simulink model "gm_zynqRadioHWSWAXI4StreamAD9361AD9364SL"  (R2024b)
settings: Solver=FixedStepDiscrete  StartTime=0.0  StopTime=18000/Fs  RelTol=1e-3
PreLoadFcn:
  | Fs = 3840000;
  | nsamp = 4096;
  | t = (0:nsamp)/Fs;
  | y = chirp(t(1:2048),0,t(2048),Fs/20,[],90);
  | ly = length(y);
InitFcn:
  | Fs = 3840000;
  | nsamp = 4096;
  | t = (0:nsamp)/Fs;
  | y = chirp(t(1:2048),0,t(2048),Fs/20,[],90);
  | ly = length(y);
libraries: hdlsllib x11, simulink x4, dspsrcs4 x2, sdrzblksprivate x1
settings Model: Creator=The MathWorks, Inc.  LastModifiedBy=daniel
settings SolverCC: AlgebraicLoopSolver=TrustRegion
settings OptimizationCC: BlockReduction=off  ConditionallyExecuteInputs=off  DefaultParameterBehavior=Inlined
settings DebuggingCC: AlgebraicLoopMsg=error  InheritedTsInSrcMsg=none  UnconnectedInputMsg=warning  UnconnectedOutputMsg=warning  UnconnectedLineMsg=warning
settings HardwareCC: ProdBitPerPointer=32  ProdBitPerSizeT=32  ProdBitPerPtrDiffT=32  ProdLargestAtomicFloat=None  ProdIntDivRoundTo=Undefined  ProdEndianess=Unspecified  ProdWordSize=32  ProdHWDeviceType=ASIC/FPGA->ASIC/FPGA  TargetBitPerLong=64  TargetBitPerPointer=64  TargetBitPerSizeT=64  TargetBitPerPtrDiffT=64  TargetLongLongMode=on  TargetIntDivRoundTo=Zero  TargetEndianess=LittleEndian  TargetWordSize=64  TargetHWDeviceType=Custom Processor->MATLAB Host Computer  ProdEqTarget=off
settings ModelReferenceCC: EnableRefExpFcnMdlSchedulingChecks=on
settings RTWCC: GPUComputeCapability=3.5

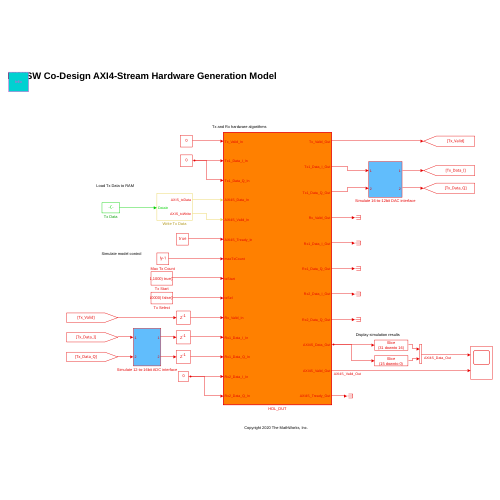
[thumbnail: Simulink's stored preview of the top-level diagram]
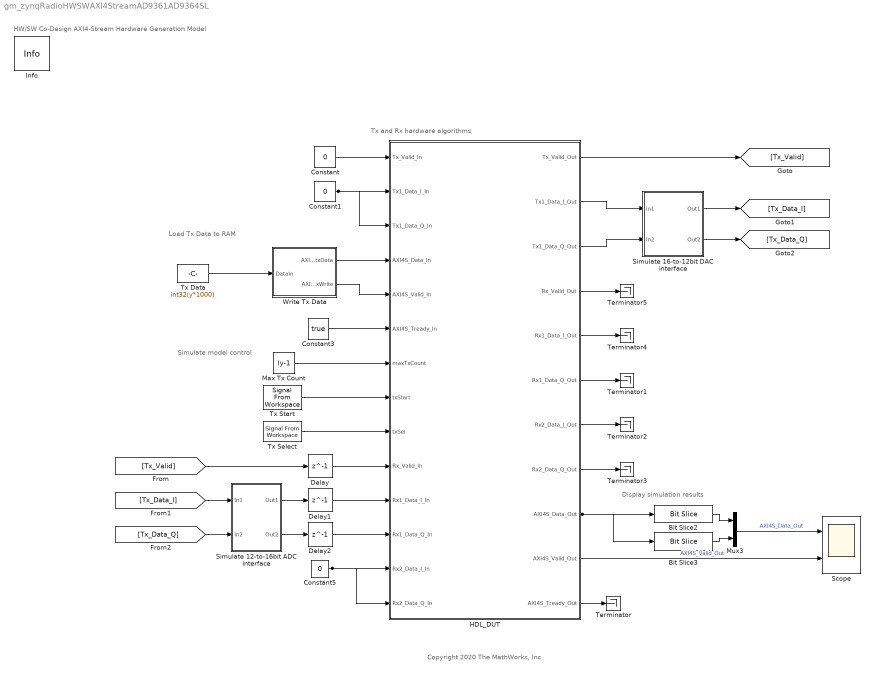
== system gm_zynqRadioHWSWAXI4StreamAD9361AD9364SL ==
  note: Copyright 2020 The MathWorks, Inc.
  note: HW/SW Co-Design AXI4-Stream Hardware Generation Model
  note: Load Tx Data to RAM
  note: Display simulation results
  note: Simulate model control
  note: Tx and Rx hardware algorithms
  Bit Slice2 : hdlsllib/Logic and Bit Operations/Bit Slice  lidx=31  ridx=16
  Bit Slice3 : hdlsllib/Logic and Bit Operations/Bit Slice  lidx=15  ridx=0
  Constant : Constant  Value=0  OutDataTypeStr=boolean  SampleTime=-1
  Constant1 : Constant  Value=0  OutDataTypeStr=int16  SampleTime=-1
  Constant3 : Constant  Value=true  SampleTime=-1
  Constant5 : Constant  Value=0  OutDataTypeStr=int16  SampleTime=-1
  Delay : Delay  DelayLength=1
  Delay1 : Delay  DelayLength=1
  Delay2 : Delay  DelayLength=1
  HDL_DUT : Subsystem  TreatAsAtomicUnit=on
  Info : sdrzblksprivate/Info  SystemSampleTime=-1  VariantActivationTime=update diagram  AllowFlexibleInterface=on  Latency=0  AutoFrameSizeCalculation=off
  Max Tx Count : Constant  Value=ly-1  OutDataTypeStr=int16  SampleTime=-1
  Mux3 : Mux  Inputs=2
  Scope : Scope  NumInputPorts=2
  Simulate 12-to-16bit ADC interface : Subsystem
  Simulate 16-to-12bit DAC interface : Subsystem
  Terminator{,1..5} (6 alike) : Terminator
  Tx Data : Constant  Value=int32(y*1000)  OutDataTypeStr=int32  SampleTime=-1
  Tx Select : dspsrcs4/Signal From Workspace  X=[true(1,10000) false(1,1000)]  Ts=1/Fs  nsamps=1  OutputAfterFinalValue=Holding final value  ignoreOrWarnInputAndFrameLengths=off  OutputFrames=off
  Tx Start : dspsrcs4/Signal From Workspace  X=[false(1,7000) true(1,100) false(1,1000) true(1,100) false(1,2000) true(1,100)]  Ts=1/Fs  nsamps=1  OutputAfterFinalValue=Setting to zero  ignoreOrWarnInputAndFrameLengths=off  OutputFrames=off
  Write Tx Data : Subsystem
  wires:
  HDL_DUT/4(Rx_Valid_Out) -> Terminator5/1
  HDL_DUT/5(Rx1_Data_I_Out) -> Terminator4/1
  HDL_DUT/8(Rx2_Data_Q_Out) -> Terminator3/1
  HDL_DUT/7(Rx2_Data_I_Out) -> Terminator2/1
  HDL_DUT/6(Rx1_Data_Q_Out) -> Terminator1/1
  Mux3/1 -> Scope/1  "AXI4S_Data_Out"
  Bit Slice3/1 -> Mux3/2
  Tx Data/1 -> Write Tx Data/1(DataIn)
  HDL_DUT/11(AXI4S_Tready_Out) -> Terminator/1
  Constant3/1 -> HDL_DUT/6(AXI4S_Tready_In)
  Simulate 12-to-16bit ADC interface/2(Out2) -> Delay2/1
  Simulate 12-to-16bit ADC interface/1(Out1) -> Delay1/1
  [Tx_Data_Q] -> Simulate 12-to-16bit ADC interface/2(In2)
  [Tx_Data_I] -> Simulate 12-to-16bit ADC interface/1(In1)
  Simulate 16-to-12bit DAC interface/2(Out2) -> [Tx_Data_Q]
  Simulate 16-to-12bit DAC interface/1(Out1) -> [Tx_Data_I]
  HDL_DUT/3(Tx1_Data_Q_Out) -> Simulate 16-to-12bit DAC interface/2(In2)
  HDL_DUT/2(Tx1_Data_I_Out) -> Simulate 16-to-12bit DAC interface/1(In1)
  HDL_DUT/9(AXI4S_Data_Out) -> Bit Slice2/1, Bit Slice3/1
  Delay/1 -> HDL_DUT/10(Rx_Valid_In)
  HDL_DUT/10(AXI4S_Valid_Out) -> Scope/2  "AXI4S_Valid_Out"
  Max Tx Count/1 -> HDL_DUT/7(maxTxCount)
  Tx Select/1 -> HDL_DUT/9(txSel)
  Tx Start/1 -> HDL_DUT/8(txStart)
  Write Tx Data/2(AXIS_txWrite) -> HDL_DUT/5(AXI4S_Valid_In)
  Constant5/1 -> HDL_DUT/14(Rx2_Data_Q_In), HDL_DUT/13(Rx2_Data_I_In)
  Constant1/1 -> HDL_DUT/3(Tx1_Data_Q_In), HDL_DUT/2(Tx1_Data_I_In)
  Write Tx Data/1(AXIS_txData) -> HDL_DUT/4(AXI4S_Data_In)
  Delay2/1 -> HDL_DUT/12(Rx1_Data_Q_In)
  Constant/1 -> HDL_DUT/1(Tx_Valid_In)
  HDL_DUT/1(Tx_Valid_Out) -> [Tx_Valid]
  Delay1/1 -> HDL_DUT/11(Rx1_Data_I_In)
  Bit Slice2/1 -> Mux3/1
  [Tx_Valid] -> Delay/1

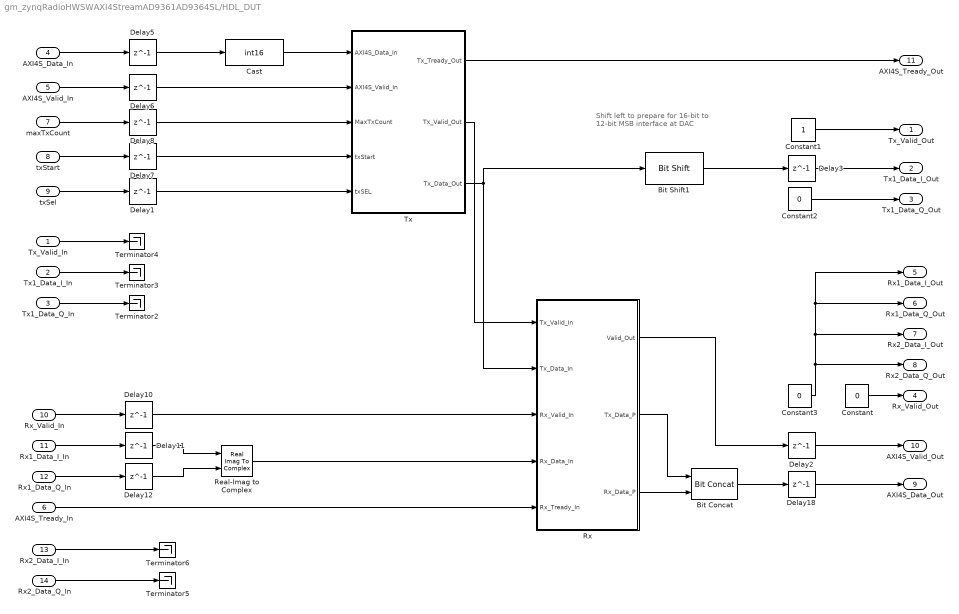
== system gm_zynqRadioHWSWAXI4StreamAD9361AD9364SL/HDL_DUT ==
  note: Shift left to prepare for 16-bit to 12-bit MSB interface at DAC
  Tx_Valid_In : Inport
  Tx1_Data_I_In : Inport  Port=2
  Tx1_Data_Q_In : Inport  Port=3
  AXI4S_Data_In : Inport  Port=4
  AXI4S_Valid_In : Inport  Port=5
  AXI4S_Tready_In : Inport  Port=6
  maxTxCount : Inport  Port=7
  txStart : Inport  Port=8
  txSel : Inport  Port=9
  Rx_Valid_In : Inport  Port=10
  Rx1_Data_I_In : Inport  Port=11
  Rx1_Data_Q_In : Inport  Port=12
  Rx2_Data_I_In : Inport  Port=13
  Rx2_Data_Q_In : Inport  Port=14
  Bit Concat : hdlsllib/Logic and Bit Operations/Bit Concat  numInputs=2
  Bit Shift1 : hdlsllib/Logic and Bit Operations/Bit Shift  mode=Shift Left Logical  N=4
  Cast : DataTypeConversion  OutDataTypeStr=int16  ConvertRealWorld=Stored Integer (SI)  SaturateOnIntegerOverflow=off  RndMeth=Floor
  Constant : Constant  Value=0  OutDataTypeStr=boolean  SampleTime=-1
  Constant1 : Constant  OutDataTypeStr=boolean  SampleTime=-1
  Constant2 : Constant  Value=0  OutDataTypeStr=int16  SampleTime=-1
  Constant3 : Constant  Value=0  OutDataTypeStr=int16  SampleTime=-1
  Delay{1..3,5..8,10..12,18} (11 alike) : Delay  DelayLength=1
  Real-Imag to Complex : RealImagToComplex
  Rx : Subsystem
  Terminator{2..6} (5 alike) : Terminator
  Tx : Subsystem
  Tx_Valid_Out : Outport
  Tx1_Data_I_Out : Outport  Port=2
  Tx1_Data_Q_Out : Outport  Port=3
  Rx_Valid_Out : Outport  Port=4
  Rx1_Data_I_Out : Outport  Port=5
  Rx1_Data_Q_Out : Outport  Port=6
  Rx2_Data_I_Out : Outport  Port=7
  Rx2_Data_Q_Out : Outport  Port=8
  AXI4S_Data_Out : Outport  Port=9
  AXI4S_Valid_Out : Outport  Port=10
  AXI4S_Tready_Out : Outport  Port=11
  wires:
  Constant1/1 -> Tx_Valid_Out/1
  Constant/1 -> Rx_Valid_Out/1
  AXI4S_Tready_In/1 -> Rx/5(Rx_Tready_In)
  Tx/1(Tx_Tready_Out) -> AXI4S_Tready_Out/1
  Delay2/1 -> AXI4S_Valid_Out/1
  Rx/3(Rx_Data_P) -> Bit Concat/2
  Rx/2(Tx_Data_P) -> Bit Concat/1
  Bit Shift1/1 -> Delay3/1
  Delay18/1 -> AXI4S_Data_Out/1
  Bit Concat/1 -> Delay18/1
  Rx/1(Valid_Out) -> Delay2/1
  Real-Imag to Complex/1 -> Rx/4(Rx_Data_In)
  Delay10/1 -> Rx/3(Rx_Valid_In)
  Constant3/1 -> Rx2_Data_Q_Out/1, Rx2_Data_I_Out/1, Rx1_Data_I_Out/1, Rx1_Data_Q_Out/1
  Constant2/1 -> Tx1_Data_Q_Out/1
  Delay3/1 -> Tx1_Data_I_Out/1
  Tx/2(Tx_Valid_Out) -> Rx/1(Tx_Valid_In)
  Delay12/1 -> Real-Imag to Complex/2
  Delay11/1 -> Real-Imag to Complex/1
  Tx/3(Tx_Data_Out) -> Rx/2(Tx_Data_In), Bit Shift1/1
  Cast/1 -> Tx/1(AXI4S_Data_In)
  Delay5/1 -> Cast/1
  Rx1_Data_Q_In/1 -> Delay12/1
  Rx1_Data_I_In/1 -> Delay11/1
  Rx_Valid_In/1 -> Delay10/1
  Rx2_Data_I_In/1 -> Terminator6/1
  Rx2_Data_Q_In/1 -> Terminator5/1
  Delay1/1 -> Tx/5(txSEL)
  Delay8/1 -> Tx/3(MaxTxCount)
  Delay7/1 -> Tx/4(txStart)
  Delay6/1 -> Tx/2(AXI4S_Valid_In)
  txSel/1 -> Delay1/1
  maxTxCount/1 -> Delay8/1
  txStart/1 -> Delay7/1
  AXI4S_Valid_In/1 -> Delay6/1
  AXI4S_Data_In/1 -> Delay5/1
  Tx1_Data_Q_In/1 -> Terminator2/1
  Tx_Valid_In/1 -> Terminator4/1
  Tx1_Data_I_In/1 -> Terminator3/1

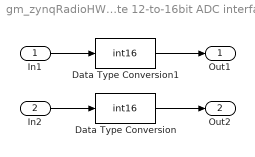
== system gm_zynqRadioHWSWAXI4StreamAD9361AD9364SL/Simulate 12-to-16bit ADC interface ==
  In1 : Inport
  In2 : Inport  Port=2
  Data Type Conversion : DataTypeConversion  OutDataTypeStr=int16  SaturateOnIntegerOverflow=off  RndMeth=Floor
  Data Type Conversion1 : DataTypeConversion  OutDataTypeStr=int16  SaturateOnIntegerOverflow=off  RndMeth=Floor
  Out1 : Outport
  Out2 : Outport  Port=2
  wires:
  Data Type Conversion/1 -> Out2/1
  In1/1 -> Data Type Conversion1/1
  Data Type Conversion1/1 -> Out1/1
  In2/1 -> Data Type Conversion/1

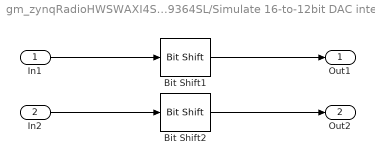
== system gm_zynqRadioHWSWAXI4StreamAD9361AD9364SL/Simulate 16-to-12bit DAC interface ==
  In1 : Inport
  In2 : Inport  Port=2
  Bit Shift1 : hdlsllib/Logic and Bit Operations/Bit Shift  mode=Shift Right Arithmetic  N=4
  Bit Shift2 : hdlsllib/Logic and Bit Operations/Bit Shift  mode=Shift Right Arithmetic  N=4
  Out1 : Outport
  Out2 : Outport  Port=2
  wires:
  Bit Shift2/1 -> Out2/1
  Bit Shift1/1 -> Out1/1
  In2/1 -> Bit Shift2/1
  In1/1 -> Bit Shift1/1

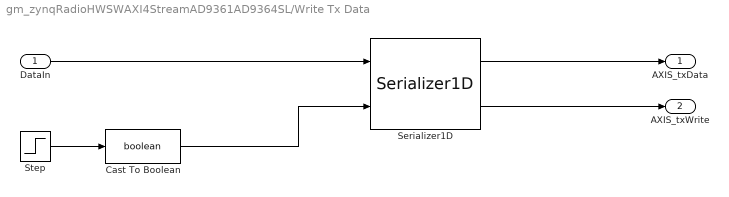
== system gm_zynqRadioHWSWAXI4StreamAD9361AD9364SL/Write Tx Data ==
  DataIn : Inport
  Cast To Boolean : DataTypeConversion  OutDataTypeStr=boolean  SaturateOnIntegerOverflow=off  RndMeth=Floor
  Serializer1D : hdlsllib/HDL Operations/Serializer1D  Ratio=2048  IdleCycles=0  validIn=on  startOut=off  validOut=on  inputDataDimensions=-1  inputSampleTime=-1  inputSignalType=auto
  Step : Step  Time=1/Fs  Before=1  After=0  SampleTime=2048/Fs
  AXIS_txData : Outport  SampleTime=1/ Fs
  AXIS_txWrite : Outport  Port=2  SampleTime=1 / Fs
  wires:
  Cast To Boolean/1 -> Serializer1D/2
  DataIn/1 -> Serializer1D/1
  Serializer1D/2 -> AXIS_txWrite/1
  Serializer1D/1 -> AXIS_txData/1
  Step/1 -> Cast To Boolean/1

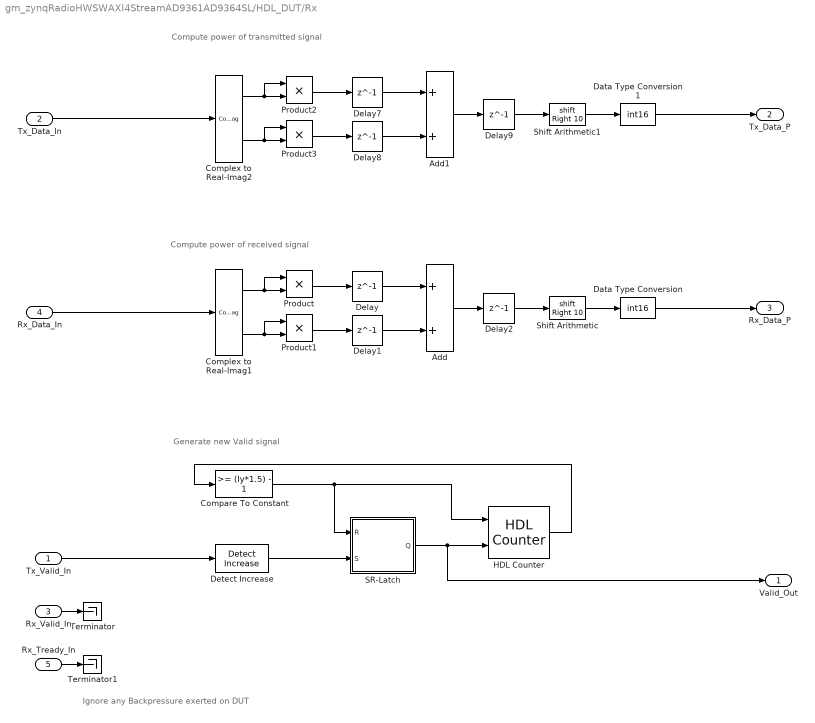
== system gm_zynqRadioHWSWAXI4StreamAD9361AD9364SL/HDL_DUT/Rx ==
  note: Compute power of transmitted signal
  note: Compute power of received signal
  note: Generate new Valid signal
  note: Ignore any Backpressure exerted on DUT
  Tx_Valid_In : Inport
  Tx_Data_In : Inport  Port=2
  Rx_Valid_In : Inport  Port=3
  Rx_Data_In : Inport  Port=4
  Rx_Tready_In : Inport  Port=5
  Add : Sum
  Add1 : Sum
  Compare To Constant : simulink/Logic and Bit Operations/Compare To Constant  relop=>=  const=(ly*1.5) - 1  OutDataTypeStr=boolean
  Complex to Real-Imag1 : ComplexToRealImag
  Complex to Real-Imag2 : ComplexToRealImag
  Data Type Conversion : DataTypeConversion  OutDataTypeStr=int16  SaturateOnIntegerOverflow=off  RndMeth=Floor
  Data Type Conversion1 : DataTypeConversion  OutDataTypeStr=int16  SaturateOnIntegerOverflow=off  RndMeth=Floor
  Delay{,1..2,7..9} (6 alike) : Delay  DelayLength=1
  Detect Increase : simulink/Logic and Bit Operations/Detect Increase  vinit=0.0  OutDataTypeStr=boolean
  HDL Counter : hdlsllib/Sources/HDL Counter  CountType=Free running  CountInit=0  CountStep=1  CountMax=(ly*1.5) - 1  CountFromType=Initial value  CountFrom=0  CountResetPort=on  CountLoadPort=off  CountEnbPort=on  CountDirPort=off  CountHitOutputPort=off  CountDataType=Unsigned  CountWordLen=12  CountFracLen=0  CountSampTime=1
  Product{,1..3} (4 alike) : Product
  SR-Latch : Subsystem
  Shift Arithmetic : ArithShift  BitShiftNumber=10  BitShiftDirection=Right
  Shift Arithmetic1 : ArithShift  BitShiftNumber=10  BitShiftDirection=Right
  Terminator : Terminator
  Terminator1 : Terminator
  Valid_Out : Outport
  Tx_Data_P : Outport  Port=2
  Rx_Data_P : Outport  Port=3
  wires:
  Rx_Tready_In/1 -> Terminator1/1
  Delay2/1 -> Shift Arithmetic/1
  Add1/1 -> Delay9/1
  Data Type Conversion1/1 -> Tx_Data_P/1
  Complex to Real-Imag2/1 -> Product2/2, Product2/1
  Delay7/1 -> Add1/1
  Delay9/1 -> Shift Arithmetic1/1
  Product2/1 -> Delay7/1
  Delay8/1 -> Add1/2
  Product3/1 -> Delay8/1
  Shift Arithmetic1/1 -> Data Type Conversion1/1
  Complex to Real-Imag2/2 -> Product3/2, Product3/1
  Tx_Data_In/1 -> Complex to Real-Imag2/1
  Rx_Data_In/1 -> Complex to Real-Imag1/1
  Data Type Conversion/1 -> Rx_Data_P/1
  Complex to Real-Imag1/1 -> Product/2, Product/1
  Delay1/1 -> Add/2
  Delay/1 -> Add/1
  Complex to Real-Imag1/2 -> Product1/2, Product1/1
  Shift Arithmetic/1 -> Data Type Conversion/1
  Product1/1 -> Delay1/1
  Add/1 -> Delay2/1
  Product/1 -> Delay/1
  Tx_Valid_In/1 -> Detect Increase/1
  SR-Latch/1(Q) -> HDL Counter/2, Valid_Out/1
  Detect Increase/1 -> SR-Latch/2(S)
  HDL Counter/1 -> Compare To Constant/1
  Compare To Constant/1 -> SR-Latch/1(R), HDL Counter/1
  Rx_Valid_In/1 -> Terminator/1

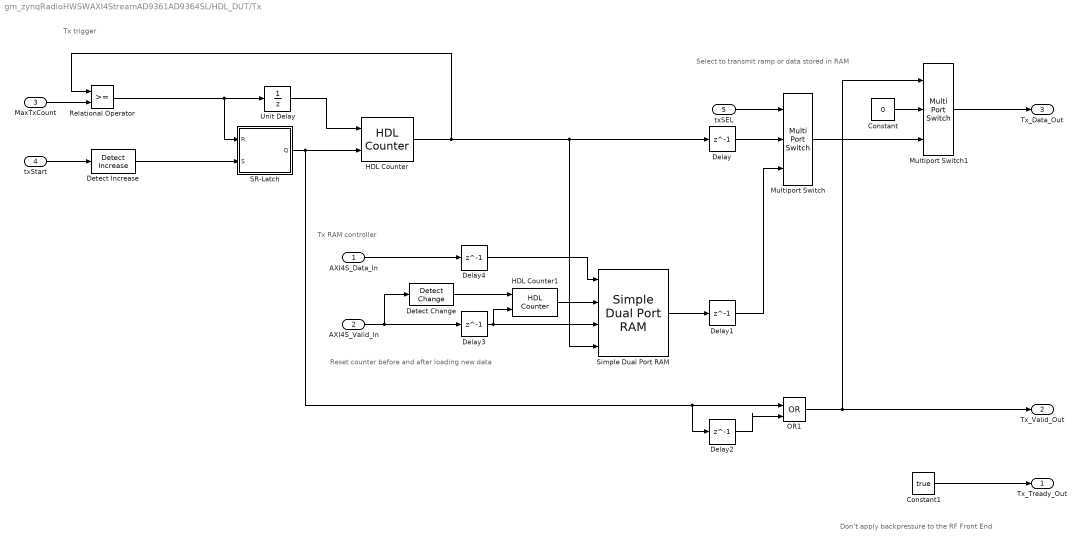
== system gm_zynqRadioHWSWAXI4StreamAD9361AD9364SL/HDL_DUT/Tx ==
  note: Don't apply backpressure to the RF Front End
  note: Tx RAM controller
  note: Tx trigger
  note: Reset counter before and after loading new data
  note: Select to transmit ramp or data stored in RAM
  AXI4S_Data_In : Inport
  AXI4S_Valid_In : Inport  Port=2
  MaxTxCount : Inport  Port=3
  txStart : Inport  Port=4
  txSEL : Inport  Port=5
  Constant : Constant  Value=0  OutDataTypeStr=int16  SampleTime=-1
  Constant1 : Constant  Value=true  SampleTime=-1
  Delay{,1..4} (5 alike) : Delay  DelayLength=1
  Detect Change : simulink/Logic and Bit Operations/Detect Change  vinit=0  OutDataTypeStr=boolean
  Detect Increase : simulink/Logic and Bit Operations/Detect Increase  vinit=0  OutDataTypeStr=boolean
  HDL Counter : hdlsllib/Sources/HDL Counter  CountType=Free running  CountInit=0  CountStep=1  CountMax=ly-1  CountFromType=Initial value  CountFrom=0  CountResetPort=on  CountLoadPort=off  CountEnbPort=on  CountDirPort=off  CountHitOutputPort=off  CountDataType=Unsigned  CountWordLen=11  CountFracLen=0  CountSampTime=1
  HDL Counter1 : hdlsllib/Sources/HDL Counter  CountType=Free running  CountInit=0  CountStep=1  CountMax=ly-1  CountFromType=Initial value  CountFrom=0  CountResetPort=on  CountLoadPort=off  CountEnbPort=on  CountDirPort=off  CountHitOutputPort=off  CountDataType=Unsigned  CountWordLen=11  CountFracLen=0  CountSampTime=1
  Multiport Switch : MultiPortSwitch  DataPortOrder=Zero-based contiguous  Inputs=2  zeroidx=on  SaturateOnIntegerOverflow=off  InputSameDT=off
  Multiport Switch1 : MultiPortSwitch  DataPortOrder=Zero-based contiguous  Inputs=2  zeroidx=on  SaturateOnIntegerOverflow=off  InputSameDT=off
  OR1 : Logic  Operator=OR  IconShape=distinctive  AllPortsSameDT=off  OutDataTypeStr=boolean
  Relational Operator : RelationalOperator  OutDataTypeStr=boolean  RndMeth=Simplest  InputSameDT=off
  SR-Latch : Subsystem
  Simple Dual Port RAM : hdlsllib/HDL RAMs/Simple Dual Port RAM  ram_size=11
  Unit Delay : UnitDelay  SampleTime=-1  HasFrameUpgradeWarning=on
  Tx_Tready_Out : Outport
  Tx_Valid_Out : Outport  Port=2
  Tx_Data_Out : Outport  Port=3
  wires:
  Constant1/1 -> Tx_Tready_Out/1
  OR1/1 -> Multiport Switch1/1, Tx_Valid_Out/1
  Constant/1 -> Multiport Switch1/2
  Delay2/1 -> OR1/2
  Multiport Switch1/1 -> Tx_Data_Out/1
  Multiport Switch/1 -> Multiport Switch1/3
  SR-Latch/1(Q) -> Delay2/1, OR1/1, HDL Counter/2
  Unit Delay/1 -> HDL Counter/1
  Delay4/1 -> Simple Dual Port RAM/1
  Delay3/1 -> HDL Counter1/2, Simple Dual Port RAM/3
  Detect Change/1 -> HDL Counter1/1
  Relational Operator/1 -> Unit Delay/1, SR-Latch/1(R)
  Delay1/1 -> Multiport Switch/3
  Delay/1 -> Multiport Switch/2
  HDL Counter1/1 -> Simple Dual Port RAM/2
  AXI4S_Data_In/1 -> Delay4/1
  txStart/1 -> Detect Increase/1
  MaxTxCount/1 -> Relational Operator/2
  txSEL/1 -> Multiport Switch/1
  HDL Counter/1 -> Relational Operator/1, Delay/1, Simple Dual Port RAM/4
  AXI4S_Valid_In/1 -> Delay3/1, Detect Change/1
  Simple Dual Port RAM/1 -> Delay1/1
  Detect Increase/1 -> SR-Latch/2(S)

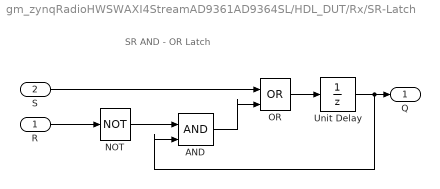
== system gm_zynqRadioHWSWAXI4StreamAD9361AD9364SL/HDL_DUT/Rx/SR-Latch ==
  note: SR AND - OR Latch
  R : Inport
  S : Inport  Port=2
  AND : Logic  IconShape=distinctive  AllPortsSameDT=off  OutDataTypeStr=boolean
  NOT : Logic  Operator=NOT  IconShape=distinctive  AllPortsSameDT=off  OutDataTypeStr=boolean
  OR : Logic  Operator=OR  IconShape=distinctive  AllPortsSameDT=off  OutDataTypeStr=boolean
  Unit Delay : UnitDelay  SampleTime=-1  HasFrameUpgradeWarning=on
  Q : Outport
  wires:
  R/1 -> NOT/1
  NOT/1 -> AND/1
  S/1 -> OR/1
  AND/1 -> OR/2
  Unit Delay/1 -> Q/1, AND/2
  OR/1 -> Unit Delay/1

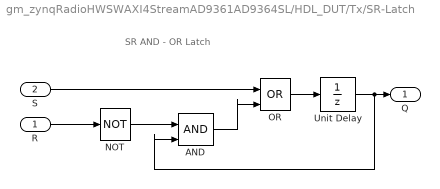
== system gm_zynqRadioHWSWAXI4StreamAD9361AD9364SL/HDL_DUT/Tx/SR-Latch ==
  note: SR AND - OR Latch
  R : Inport
  S : Inport  Port=2
  AND : Logic  IconShape=distinctive  AllPortsSameDT=off  OutDataTypeStr=boolean
  NOT : Logic  Operator=NOT  IconShape=distinctive  AllPortsSameDT=off  OutDataTypeStr=boolean
  OR : Logic  Operator=OR  IconShape=distinctive  AllPortsSameDT=off  OutDataTypeStr=boolean
  Unit Delay : UnitDelay  SampleTime=-1  HasFrameUpgradeWarning=on
  Q : Outport
  wires:
  R/1 -> NOT/1
  NOT/1 -> AND/1
  S/1 -> OR/1
  AND/1 -> OR/2
  Unit Delay/1 -> Q/1, AND/2
  OR/1 -> Unit Delay/1
